simulink model "WEEK1_QN1"  (R2020b)
settings: Solver=VariableStepAuto  StartTime=0.0  StopTime=10.0  MaxStep=0.001  RelTol=1e-3
model workspace (MAT data in the model file):
  K1 = 50
  K12 = 5000
  M1 = 100
  M2 = 50
  Sig = Simulink.Signal
  Sig.DataType = 'auto'
  Sig.Dimensions = -1
  Sig.DimensionsMode = 'auto'
  Sig.Complexity = 'auto'
  Sig.SampleTime = -1
  Sig.SamplingMode = 'auto'
  b = 50
settings Model: Creator=dell  LastModifiedBy=dell

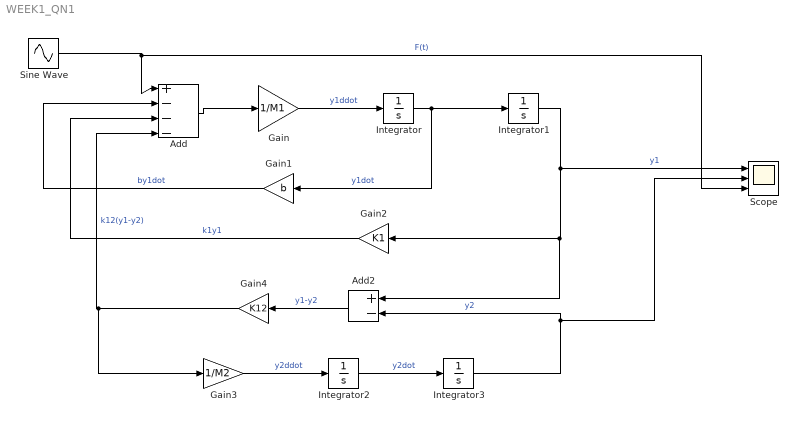
== system WEEK1_QN1 ==
  Add : Sum  Inputs=+---
  Add2 : Sum  Inputs=+-
  Gain : Gain  Gain=1/M1
  Gain1 : Gain  Gain=b
  Gain2 : Gain  Gain=K1
  Gain3 : Gain  Gain=1/M2
  Gain4 : Gain  Gain=K12
  Integrator{,1..3} (4 alike) : Integrator
  Scope : Scope  NumInputPorts=3
  Sine Wave : Sin  Amplitude=2  Frequency=10  SampleTime=0
  wires:
  Gain3/1 -> Integrator2/1  "y2ddot"
  Gain4/1 -> Gain3/1, Add/4  "k12(y1-y2)"
  Gain2/1 -> Add/3  "k1y1"
  Gain1/1 -> Add/2  "by1dot"
  Add/1 -> Gain/1
  Integrator1/1 -> Add2/1, Gain2/1, Scope/1  "y1"
  Gain/1 -> Integrator/1  "y1ddot"
  Integrator/1 -> Gain1/1, Integrator1/1  "y1dot"
  Integrator3/1 -> Scope/2, Add2/2  "y2"
  Integrator2/1 -> Integrator3/1  "y2dot"
  Sine Wave/1 -> Scope/3, Add/1  "F(t)"
  Add2/1 -> Gain4/1  "y1-y2"
